simulink model "AppDesignerWithSimulink"  (R2018b)
settings: Solver=VariableStepAuto  StartTime=0.0  StopTime=inf  RelTol=1e-3
model workspace (MAT data in the model file):
  A = 0
  OFF = 0
  ON = 1
settings Model: EnablePacing=on  Creator=lmerid1  LastModifiedBy=lmerid1

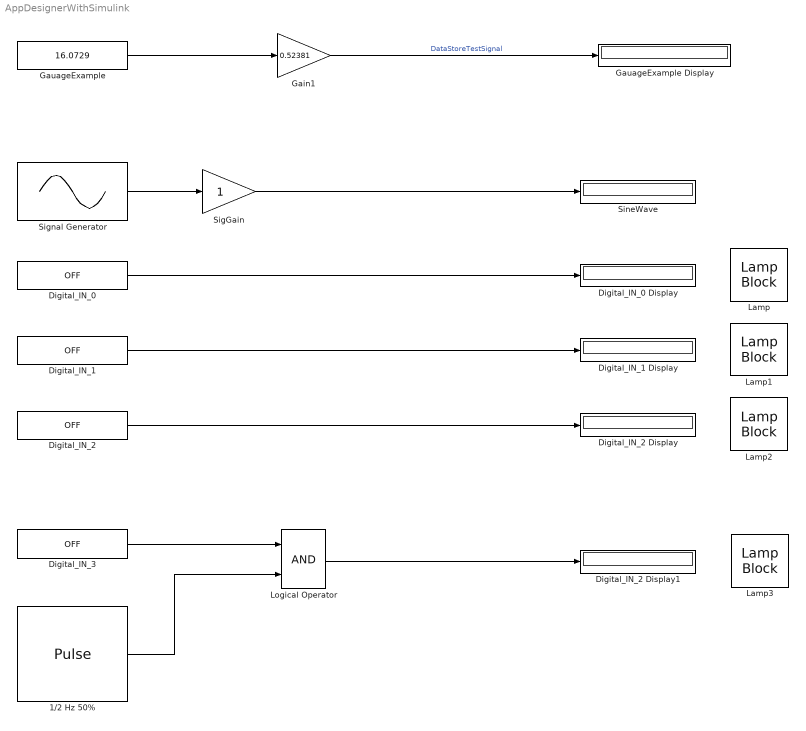
== system AppDesignerWithSimulink ==
  1/2 Hz 50% : DiscretePulseGenerator  PulseType=Time based  PulseWidth=50
  Digital_IN_{0..3} (4 alike) : Constant  Value=OFF
  Digital_IN_0 Display : Display
  Digital_IN_1 Display : Display
  Digital_IN_2 Display : Display
  Digital_IN_2 Display1 : Display
  Gain1 : Gain  Gain=0.52381
  GauageExample : Constant  Value=16.0729
  GauageExample Display : Display
  Lamp : LampBlock  WebBlockId=21  LabelPosition=Hide
  Lamp1 : LampBlock  WebBlockId=25  LabelPosition=Hide
  Lamp2 : LampBlock  WebBlockId=26  LabelPosition=Hide
  Lamp3 : LampBlock  WebBlockId=38  LabelPosition=Hide
  Logical Operator : Logic  AllPortsSameDT=off  OutDataTypeStr=boolean
  SigGain : Gain
  Signal Generator : Sin  SampleTime=0
  SineWave : Display
  wires:
  Digital_IN_0/1 -> Digital_IN_0 Display/1
  Digital_IN_2/1 -> Digital_IN_2 Display/1
  Digital_IN_1/1 -> Digital_IN_1 Display/1
  GauageExample/1 -> Gain1/1
  Digital_IN_3/1 -> Logical Operator/1
  1/2 Hz 50%/1 -> Logical Operator/2
  Logical Operator/1 -> Digital_IN_2 Display1/1
  Signal Generator/1 -> SigGain/1
  SigGain/1 -> SineWave/1
  Gain1/1 -> GauageExample Display/1  "DataStoreTestSignal"
